simulink model "PID_conventional"  (R2025b)
settings: Solver=FixedStepAuto  StartTime=0.0  StopTime=150.0  FixedStep=1e-3  RelTol=1e-3
undefined symbols (not defined in the file or in its folder): Kp, Td, Tf, Ti
settings Model: Creator=Uros  LastModifiedBy=Uros
settings ModelReferenceCC: ModelReferenceMinAlgLoopOccurrences=on

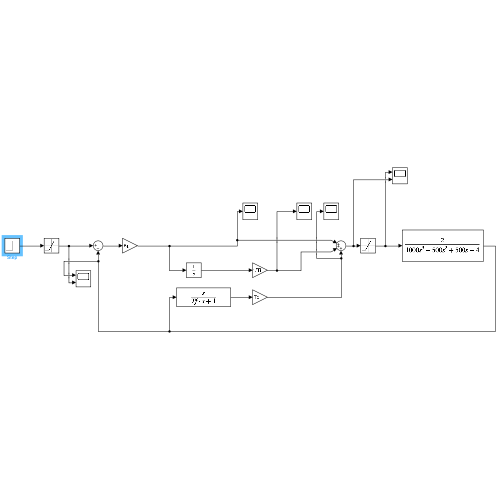
[thumbnail: Simulink's stored preview of the top-level diagram]
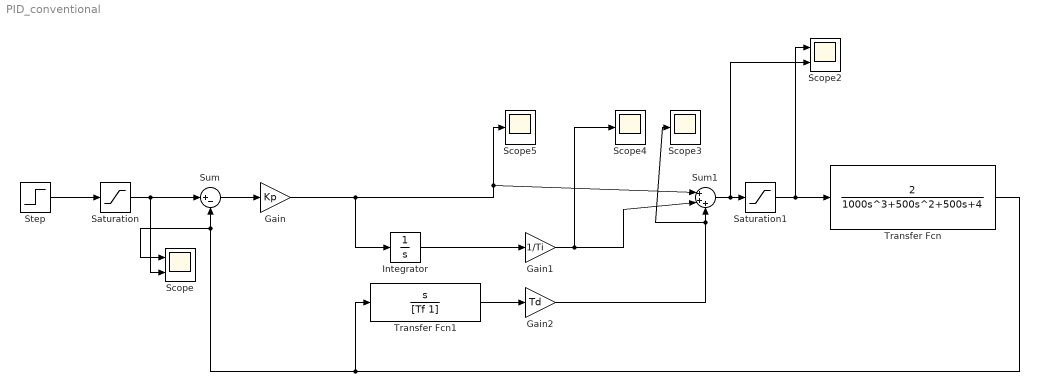
== system PID_conventional ==
  Gain : Gain  Gain=Kp
  Gain1 : Gain  Gain=1/Ti
  Gain2 : Gain  Gain=Td
  Integrator : Integrator
  Saturation : Saturate  UpperLimit=3  LowerLimit=-3
  Saturation1 : Saturate  UpperLimit=15  LowerLimit=-15
  Scope : Scope  NumInputPorts=2
      settings: ActiveDisplayYMinimum=-0.44433279742765275  ActiveDisplayYMaximum=3.493167202572347
  Scope2 : Scope  NumInputPorts=2
      settings: ActiveDisplayYMinimum=-14.460291854058777  ActiveDisplayYMaximum=85.902623082247814  DataLoggingVariableName=ScopeData2
  Scope3 : Scope
      settings: ActiveDisplayYMinimum=-2.8765238422338411  ActiveDisplayYMaximum=3.2803438957612743  DataLoggingVariableName=ScopeData3
  Scope4 : Scope
      settings: ActiveDisplayYMinimum=-8.43713582868526  ActiveDisplayYMaximum=75.934222458167355  DataLoggingVariableName=ScopeData4
  Scope5 : Scope
      settings: ActiveDisplayYMinimum=-32.590620337805888  ActiveDisplayYMaximum=53.621180037533989  DataLoggingVariableName=ScopeData5
  Step : Step  Time=10  After=5  SampleTime=0
  Sum : Sum  Inputs=|+-
  Sum1 : Sum  Inputs=|+++
  Transfer Fcn : TransferFcn  Numerator=[2]  Denominator=[1000 500 500 4]
  Transfer Fcn1 : TransferFcn  Numerator=[1 0]  Denominator=[Tf 1]
  wires:
  Transfer Fcn/1 -> Transfer Fcn1/1, Scope/1, Sum/2
  Transfer Fcn1/1 -> Gain2/1
  Gain1/1 -> Sum1/2, Scope4/1
  Gain2/1 -> Scope3/1, Sum1/3
  Integrator/1 -> Gain1/1
  Step/1 -> Saturation/1
  Saturation/1 -> Scope/2, Sum/1
  Sum1/1 -> Scope2/2, Saturation1/1
  Saturation1/1 -> Scope2/1, Transfer Fcn/1
  Sum/1 -> Gain/1
  Gain/1 -> Integrator/1, Scope5/1, Sum1/1
